simulink model "accTests"  (R2019a)
settings: Solver=VariableStepAuto  StartTime=0.0  StopTime=20  RelTol=1e-3
values from neighbouring files (symbols this model uses):
  ehMax = 3    [sim_parameters.m]
  ehMin = -100    [sim_parameters.m]
  g0 = 1/2*maxAccel*T^2 + maxAccel*T*t1 + + 1/2*maxAccel*t1^2 + 1/6*minJerk*t1^3 -      1/(2*minAccel)*(maxAccel*T + maxAccel*t1+ 1/2*minJerk*t1^2)^2    [safeHeadway.m]    (also in sim_parameters.m = ceil(g0*10)*1.1/10)
  h = figure()    [plotKinematicsFromSimulink.m]    (also in safeHeadway.m = T + t1 -      1/minAccel*(maxAccel*T + maxAccel*t1+1/2*minJe; sim_parameters.m = ceil(h*10)*1.1/10)
  Kd = K(1)    [SimulinkScenario.m]
  Ki = K(3)    [SimulinkScenario.m]
  Kp = K(2)    [SimulinkScenario.m]
  maxAcc = 4    [sim_parameters.m]
  maxJerk = 40    [sim_parameters.m]
  minAcc = -8    [sim_parameters.m]
  minJerk = -75    [sim_parameters.m]
  p = 10    [sim_parameters.m]
  vehMass = 2000    [sim_parameters.m]
  vLen = lf+lr    (= 3)    [sim_parameters.m]
libraries: autolibshared x5
settings Model: Creator=Fernando VM  LastModifiedBy=fvall
settings DataIOCC: ReturnWorkspaceOutputs=off
settings DebuggingCC: ArithmeticOperatorsInVariantConditions=warning

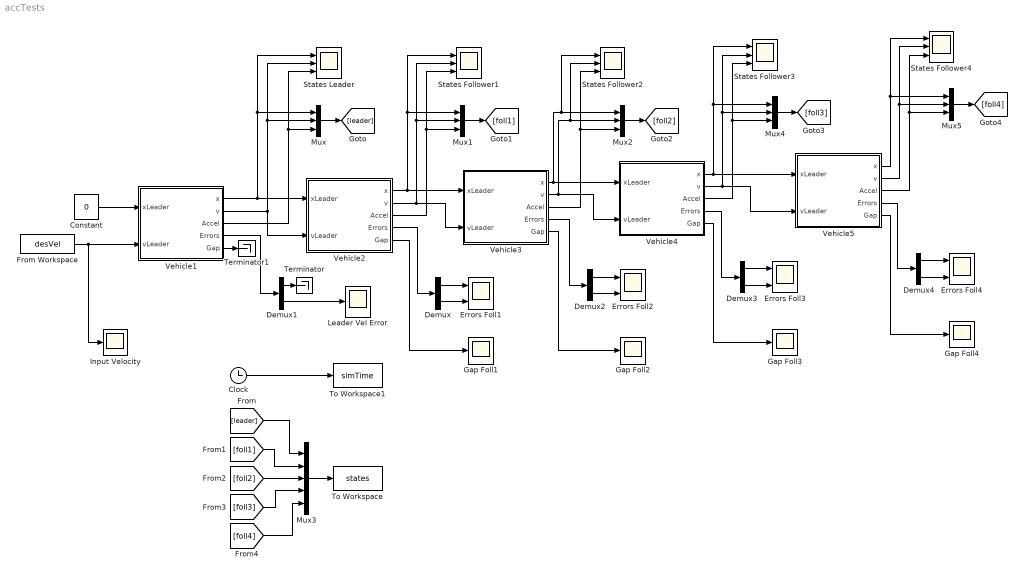
== system accTests ==
  Clock : Clock
  Constant : Constant  Value=0
  Demux{,1..4} (5 alike) : Demux  Outputs=2
  Errors Foll{1..4} (4 alike) : Scope  NumInputPorts=2
  From Workspace : FromWorkspace  VariableName=desVel  SampleTime=0
  Gap Foll{1..4} (4 alike) : Scope
  Input Velocity : Scope
  Leader Vel Error : Scope
  Mux{,1..2,4..5} (5 alike) : Mux  Inputs=3
  Mux3 : Mux  Inputs=5
  States Follower{1..4} (4 alike) : Scope  NumInputPorts=3
  States Leader : Scope  NumInputPorts=3
  Terminator : Terminator
  Terminator1 : Terminator
  To Workspace : ToWorkspace  VariableName=states  SampleTime=-1
  To Workspace1 : ToWorkspace  VariableName=simTime  SampleTime=-1
  Vehicle1 : Subsystem  mask{vehMass=vehMass, vLen=vLen, maxAcceleration=maxAcc, minAcceleration=minAcc, maxJerk=maxJerk, minJerk=minJerk, X_o=12.44, initVel=0, Kp=Kp, Kd=Kd, Ki=Ki, h=h, g0=g0, minHeadwayError=ehMin, maxHeadwayError=ehMax, velFilterGain=p}
      mask prompts: vehMass "Vehicle Mass"; vLen "Vehicle Length"; maxAcceleration "Max Acceleration"; minAcceleration "Min Acceleration"; maxJerk "Max Jerk"; minJerk "Min Jerk"; X_o "Initial Longitudinal Position"; initVel "Initial Longitudinal Velocity"; h "Time Headway"; g0 "Standstill Gap"; minHeadwayError "Min Headway Error"; maxHeadwayError "Max Headway Error"; velFilterGain "Velocity Filter Gain"
      mask DialogControl DescGroupVar Prompt: 3DOF Vehicle with ACC
      mask DialogControl DescTextVar Prompt: Vehicle with ACC. The vehicle model is Simulink's 3DOF single track vehicle body. The controller is a PID with constant headway including headway error saturation and filtered leader velocity.
      mask DialogControl ParameterGroupVar Prompt: Vehicle Parameters
      mask DialogControl Container3 Prompt: Controller Parameters
  Vehicle2 : Subsystem  mask{vehMass=vehMass, vLen=vLen, maxAcceleration=maxAcc, minAcceleration=minAcc, maxJerk=maxJerk, minJerk=minJerk, X_o=9.33, initVel=0, Kp=Kp, Kd=Kd, Ki=Ki, h=h, g0=g0, minHeadwayError=ehMin, maxHeadwayError=ehMax, velFilterGain=p}
      mask prompts: vehMass "Vehicle Mass"; vLen "Vehicle Length"; maxAcceleration "Max Acceleration"; minAcceleration "Min Acceleration"; maxJerk "Max Jerk"; minJerk "Min Jerk"; X_o "Initial Longitudinal Position"; initVel "Initial Longitudinal Velocity"; h "Time Headway"; g0 "Standstill Gap"; minHeadwayError "Min Headway Error"; maxHeadwayError "Max Headway Error"; velFilterGain "Velocity Filter Gain"
      mask DialogControl DescGroupVar Prompt: 3DOF Vehicle with ACC
      mask DialogControl DescTextVar Prompt: Vehicle with ACC. The vehicle model is Simulink's 3DOF single track vehicle body. The controller is a PID with constant headway including headway error saturation and filtered leader velocity.
      mask DialogControl ParameterGroupVar Prompt: Vehicle Parameters
      mask DialogControl Container3 Prompt: Controller Parameters
  Vehicle3 : Subsystem  mask{vehMass=vehMass, vLen=vLen, maxAcceleration=maxAcc, minAcceleration=minAcc, maxJerk=maxJerk, minJerk=minJerk, X_o=6.22, initVel=0, Kp=Kp, Kd=Kd, Ki=Ki, h=h, g0=g0, minHeadwayError=ehMin, maxHeadwayError=ehMax, velFilterGain=p}
      mask prompts: vehMass "Vehicle Mass"; vLen "Vehicle Length"; maxAcceleration "Max Acceleration"; minAcceleration "Min Acceleration"; maxJerk "Max Jerk"; minJerk "Min Jerk"; X_o "Initial Longitudinal Position"; initVel "Initial Longitudinal Velocity"; h "Time Headway"; g0 "Standstill Gap"; minHeadwayError "Min Headway Error"; maxHeadwayError "Max Headway Error"; velFilterGain "Velocity Filter Gain"
      mask DialogControl DescGroupVar Prompt: 3DOF Vehicle with ACC
      mask DialogControl DescTextVar Prompt: Vehicle with ACC. The vehicle model is Simulink's 3DOF single track vehicle body. The controller is a PID with constant headway including headway error saturation and filtered leader velocity.
      mask DialogControl ParameterGroupVar Prompt: Vehicle Parameters
      mask DialogControl Container3 Prompt: Controller Parameters
  Vehicle4 : Subsystem  mask{vehMass=vehMass, vLen=vLen, maxAcceleration=maxAcc, minAcceleration=minAcc, maxJerk=maxJerk, minJerk=minJerk, X_o=3.11, initVel=0, Kp=Kp, Kd=Kd, Ki=Ki, h=h, g0=g0, minHeadwayError=ehMin, maxHeadwayError=ehMax, velFilterGain=p}
      mask prompts: vehMass "Vehicle Mass"; vLen "Vehicle Length"; maxAcceleration "Max Acceleration"; minAcceleration "Min Acceleration"; maxJerk "Max Jerk"; minJerk "Min Jerk"; X_o "Initial Longitudinal Position"; initVel "Initial Longitudinal Velocity"; h "Time Headway"; g0 "Standstill Gap"; minHeadwayError "Min Headway Error"; maxHeadwayError "Max Headway Error"; velFilterGain "Velocity Filter Gain"
      mask DialogControl DescGroupVar Prompt: 3DOF Vehicle with ACC
      mask DialogControl DescTextVar Prompt: Vehicle with ACC. The vehicle model is Simulink's 3DOF single track vehicle body. The controller is a PID with constant headway including headway error saturation and filtered leader velocity.
      mask DialogControl ParameterGroupVar Prompt: Vehicle Parameters
      mask DialogControl Container3 Prompt: Controller Parameters
  Vehicle5 : Subsystem  mask{vehMass=vehMass, vLen=vLen, maxAcceleration=maxAcc, minAcceleration=minAcc, maxJerk=maxJerk, minJerk=minJerk, X_o=0, initVel=0, Kp=Kp, Kd=Kd, Ki=Ki, h=h, g0=g0, minHeadwayError=ehMin, maxHeadwayError=ehMax, velFilterGain=p}
      mask prompts: vehMass "Vehicle Mass"; vLen "Vehicle Length"; maxAcceleration "Max Acceleration"; minAcceleration "Min Acceleration"; maxJerk "Max Jerk"; minJerk "Min Jerk"; X_o "Initial Longitudinal Position"; initVel "Initial Longitudinal Velocity"; h "Time Headway"; g0 "Standstill Gap"; minHeadwayError "Min Headway Error"; maxHeadwayError "Max Headway Error"; velFilterGain "Velocity Filter Gain"
      mask DialogControl DescGroupVar Prompt: 3DOF Vehicle with ACC
      mask DialogControl DescTextVar Prompt: Vehicle with ACC. The vehicle model is Simulink's 3DOF single track vehicle body. The controller is a PID with constant headway including headway error saturation and filtered leader velocity.
      mask DialogControl ParameterGroupVar Prompt: Vehicle Parameters
      mask DialogControl Container3 Prompt: Controller Parameters
  wires:
  Vehicle2/5(Gap) -> Gap Foll1/1
  Vehicle5/3(Accel) -> Mux5/3, States Follower4/3
  Vehicle3/4(Errors) -> Demux2/1
  Vehicle3/1(x) -> Vehicle4/1(xLeader), Mux2/1, States Follower2/1
  Demux2/1 -> Errors Foll2/1
  Demux4/1 -> Errors Foll4/1
  Clock/1 -> To Workspace1/1
  Vehicle5/5(Gap) -> Gap Foll4/1
  Vehicle4/1(x) -> Vehicle5/1(xLeader), Mux4/1, States Follower3/1
  Vehicle4/3(Accel) -> Mux4/3, States Follower3/3
  Vehicle1/4(Errors) -> Demux1/1
  Demux/1 -> Errors Foll1/1
  Constant/1 -> Vehicle1/1(xLeader)
  Vehicle4/5(Gap) -> Gap Foll3/1
  Vehicle4/2(v) -> Vehicle5/2(vLeader), Mux4/2, States Follower3/2
  Mux4/1 -> [foll3]
  Vehicle2/1(x) -> Vehicle3/1(xLeader), Mux1/1, States Follower1/1
  Vehicle2/4(Errors) -> Demux/1
  Vehicle5/4(Errors) -> Demux4/1
  Vehicle3/2(v) -> Vehicle4/2(vLeader), Mux2/2, States Follower2/2
  Mux5/1 -> [foll4]
  Vehicle4/4(Errors) -> Demux3/1
  [foll1] -> Mux3/2
  Vehicle5/2(v) -> Mux5/2, States Follower4/2
  Demux4/2 -> Errors Foll4/2
  Vehicle1/1(x) -> Vehicle2/1(xLeader), States Leader/1, Mux/1
  Demux/2 -> Errors Foll1/2
  [foll3] -> Mux3/4
  [foll4] -> Mux3/5
  Mux3/1 -> To Workspace/1
  Mux2/1 -> [foll2]
  [leader] -> Mux3/1
  Mux1/1 -> [foll1]
  Mux/1 -> [leader]
  Demux2/2 -> Errors Foll2/2
  Vehicle2/2(v) -> Vehicle3/2(vLeader), Mux1/2, States Follower1/2
  [foll2] -> Mux3/3
  Vehicle2/3(Accel) -> Mux1/3, States Follower1/3
  Vehicle3/5(Gap) -> Gap Foll2/1
  Demux3/2 -> Errors Foll3/2
  Vehicle1/5(Gap) -> Terminator1/1
  Vehicle1/3(Accel) -> States Leader/3, Mux/3
  Demux1/2 -> Leader Vel Error/1
  Demux3/1 -> Errors Foll3/1
  Vehicle3/3(Accel) -> Mux2/3, States Follower2/3
  From Workspace/1 -> Input Velocity/1, Vehicle1/2(vLeader)
  Demux1/1 -> Terminator/1
  Vehicle1/2(v) -> Vehicle2/2(vLeader), Mux/2, States Leader/2
  Vehicle5/1(x) -> Mux5/1, States Follower4/1

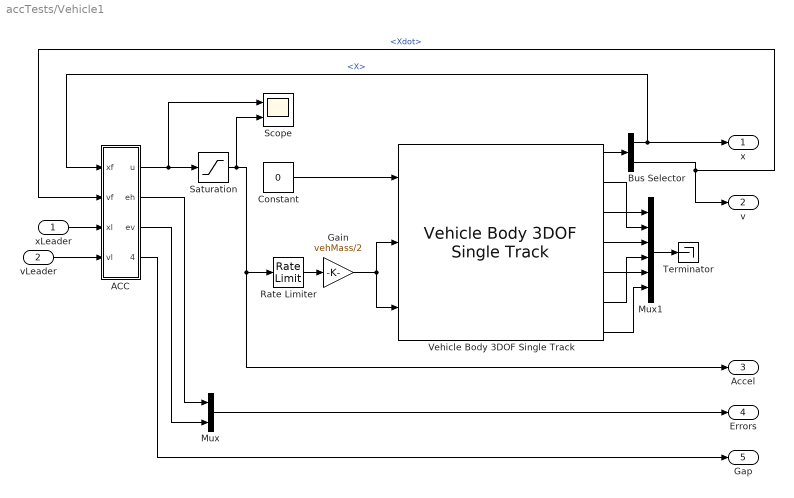
== system accTests/Vehicle1 ==
  xLeader : Inport
  vLeader : Inport  Port=2
  ACC : Subsystem
  Bus Selector : BusSelector  OutputSignals=InertFrm.RearAxl.Disp.X,InertFrm.RearAxl.Vel.Xdot
  Constant : Constant  Value=0
  Gain : Gain  Gain=vehMass/2
  Mux : Mux  Inputs=2
  Mux1 : Mux  Inputs=6
  Rate Limiter : RateLimiter  RisingSlewLimit=maxJerk  FallingSlewLimit=minJerk  SampleTimeMode=inherited
  Saturation : Saturate  UpperLimit=maxAcc  LowerLimit=minAcc
  Scope : Scope  NumInputPorts=2
  Terminator : Terminator
  Vehicle Body 3DOF Single Track : autolibshared/Vehicle Body 3DOF Single Track  trackMode=Single (bicycle)  inputMode=External longitudinal forces  frontSteerMode=on  rearSteerMode=off  windMode=off  muMode=off  extFMode=off  extMMode=off  extXo=off  extpsio=off  extxdoto=off  extro=off  extYo=off  extTamb=off  extydoto=off  aMode=2  NF=2  NR=2  m=vehMass  a=vLen/2  b=vLen/2  h=0.35  X_o=X_o  xdot_o=initVel  CalphaMode=off  sigmaMode=on  d=0  w=[1.4,1.4]  Cy_f=12e3  Cy_r=11e3  sigma_f=.1  sigma_r=.1  alpha_f_brk=[-.1 .1]  Cy_f_data=[-9e3 9e3]  alpha_r_brk=[-.1 .1]  Cy_r_data=[-9e3 9e3]  Y_o=0  ydot_o=0  Izz=4000  psi_o=0  r_o=0  Af=2  Cd=.3  Cl=.1  Cpm=.1  beta_w=[0:0.01:0.3]  Cs=[0:0.03:0.9]  Cym=[0:0.01:0.3]  Pabs=101325  Tair=273  g=9.81  mu=1  xdot_tol=.01  Fznom=5000  Fxtire_sat=7e4  Fytire_sat=7e4  longOff=0  latOff=0  vertOff=0  wrapAng=off
      settings: SourceProductName=Powertrain Blockset  SourceProductBaseCode=PW
  x : Outport
  v : Outport  Port=2
  Accel : Outport  Port=3
  Errors : Outport  Port=4
  Gap : Outport  Port=5
  wires:
  Bus Selector/2 -> ACC/2(vf), v/1  "<Xdot>"
  Bus Selector/1 -> x/1, ACC/1(xf)  "<X>"
  Saturation/1 -> Scope/2, Rate Limiter/1, Accel/1
  vLeader/1 -> ACC/4(vl)
  ACC/1(u) -> Scope/1, Saturation/1
  xLeader/1 -> ACC/3(xl)
  ACC/2(eh) -> Mux/1
  ACC/3(ev) -> Mux/2
  Mux/1 -> Errors/1
  Gain/1 -> Vehicle Body 3DOF Single Track/2, Vehicle Body 3DOF Single Track/3
  Constant/1 -> Vehicle Body 3DOF Single Track/1
  Vehicle Body 3DOF Single Track/1 -> Bus Selector/1
  Vehicle Body 3DOF Single Track/4 -> Mux1/3
  Vehicle Body 3DOF Single Track/3 -> Mux1/2
  Vehicle Body 3DOF Single Track/2 -> Mux1/1
  Vehicle Body 3DOF Single Track/5 -> Mux1/4
  Vehicle Body 3DOF Single Track/6 -> Mux1/5
  Vehicle Body 3DOF Single Track/7 -> Mux1/6
  Mux1/1 -> Terminator/1
  ACC/4(gap) -> Gap/1
  Rate Limiter/1 -> Gain/1

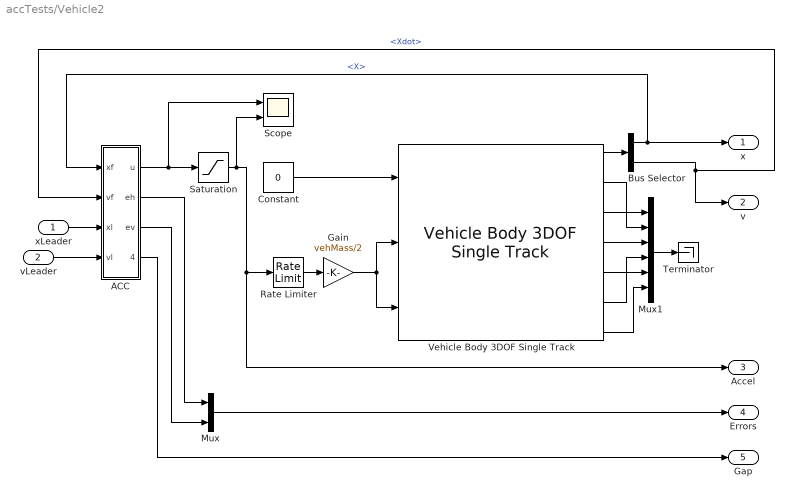
== system accTests/Vehicle2 ==
  xLeader : Inport
  vLeader : Inport  Port=2
  ACC : Subsystem
  Bus Selector : BusSelector  OutputSignals=InertFrm.RearAxl.Disp.X,InertFrm.RearAxl.Vel.Xdot
  Constant : Constant  Value=0
  Gain : Gain  Gain=vehMass/2
  Mux : Mux  Inputs=2
  Mux1 : Mux  Inputs=6
  Rate Limiter : RateLimiter  RisingSlewLimit=maxJerk  FallingSlewLimit=minJerk  SampleTimeMode=inherited
  Saturation : Saturate  UpperLimit=maxAcc  LowerLimit=minAcc
  Scope : Scope  NumInputPorts=2
  Terminator : Terminator
  Vehicle Body 3DOF Single Track : autolibshared/Vehicle Body 3DOF Single Track  trackMode=Single (bicycle)  inputMode=External longitudinal forces  frontSteerMode=on  rearSteerMode=off  windMode=off  muMode=off  extFMode=off  extMMode=off  extXo=off  extpsio=off  extxdoto=off  extro=off  extYo=off  extTamb=off  extydoto=off  aMode=2  NF=2  NR=2  m=vehMass  a=vLen/2  b=vLen/2  h=0.35  X_o=X_o  xdot_o=initVel  CalphaMode=off  sigmaMode=on  d=0  w=[1.4,1.4]  Cy_f=12e3  Cy_r=11e3  sigma_f=.1  sigma_r=.1  alpha_f_brk=[-.1 .1]  Cy_f_data=[-9e3 9e3]  alpha_r_brk=[-.1 .1]  Cy_r_data=[-9e3 9e3]  Y_o=0  ydot_o=0  Izz=4000  psi_o=0  r_o=0  Af=2  Cd=.3  Cl=.1  Cpm=.1  beta_w=[0:0.01:0.3]  Cs=[0:0.03:0.9]  Cym=[0:0.01:0.3]  Pabs=101325  Tair=273  g=9.81  mu=1  xdot_tol=.01  Fznom=5000  Fxtire_sat=7e4  Fytire_sat=7e4  longOff=0  latOff=0  vertOff=0  wrapAng=off
      settings: SourceProductName=Powertrain Blockset  SourceProductBaseCode=PW
  x : Outport
  v : Outport  Port=2
  Accel : Outport  Port=3
  Errors : Outport  Port=4
  Gap : Outport  Port=5
  wires:
  Bus Selector/2 -> ACC/2(vf), v/1  "<Xdot>"
  Bus Selector/1 -> x/1, ACC/1(xf)  "<X>"
  Saturation/1 -> Scope/2, Rate Limiter/1, Accel/1
  vLeader/1 -> ACC/4(vl)
  ACC/1(u) -> Scope/1, Saturation/1
  xLeader/1 -> ACC/3(xl)
  ACC/2(eh) -> Mux/1
  ACC/3(ev) -> Mux/2
  Mux/1 -> Errors/1
  Gain/1 -> Vehicle Body 3DOF Single Track/2, Vehicle Body 3DOF Single Track/3
  Constant/1 -> Vehicle Body 3DOF Single Track/1
  Vehicle Body 3DOF Single Track/1 -> Bus Selector/1
  Vehicle Body 3DOF Single Track/4 -> Mux1/3
  Vehicle Body 3DOF Single Track/3 -> Mux1/2
  Vehicle Body 3DOF Single Track/2 -> Mux1/1
  Vehicle Body 3DOF Single Track/5 -> Mux1/4
  Vehicle Body 3DOF Single Track/6 -> Mux1/5
  Vehicle Body 3DOF Single Track/7 -> Mux1/6
  Mux1/1 -> Terminator/1
  ACC/4(gap) -> Gap/1
  Rate Limiter/1 -> Gain/1

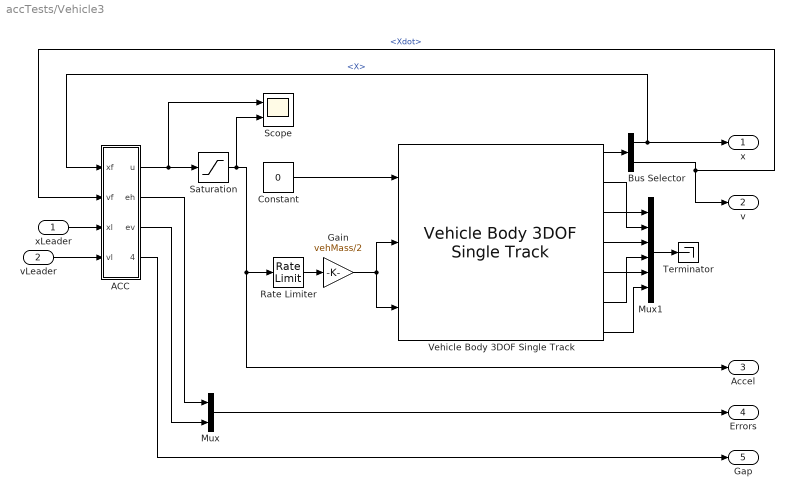
== system accTests/Vehicle3 ==
  xLeader : Inport
  vLeader : Inport  Port=2
  ACC : Subsystem
  Bus Selector : BusSelector  OutputSignals=InertFrm.RearAxl.Disp.X,InertFrm.RearAxl.Vel.Xdot
  Constant : Constant  Value=0
  Gain : Gain  Gain=vehMass/2
  Mux : Mux  Inputs=2
  Mux1 : Mux  Inputs=6
  Rate Limiter : RateLimiter  RisingSlewLimit=maxJerk  FallingSlewLimit=minJerk  SampleTimeMode=inherited
  Saturation : Saturate  UpperLimit=maxAcc  LowerLimit=minAcc
  Scope : Scope  NumInputPorts=2
  Terminator : Terminator
  Vehicle Body 3DOF Single Track : autolibshared/Vehicle Body 3DOF Single Track  trackMode=Single (bicycle)  inputMode=External longitudinal forces  frontSteerMode=on  rearSteerMode=off  windMode=off  muMode=off  extFMode=off  extMMode=off  extXo=off  extpsio=off  extxdoto=off  extro=off  extYo=off  extTamb=off  extydoto=off  aMode=2  NF=2  NR=2  m=vehMass  a=vLen/2  b=vLen/2  h=0.35  X_o=X_o  xdot_o=initVel  CalphaMode=off  sigmaMode=on  d=0  w=[1.4,1.4]  Cy_f=12e3  Cy_r=11e3  sigma_f=.1  sigma_r=.1  alpha_f_brk=[-.1 .1]  Cy_f_data=[-9e3 9e3]  alpha_r_brk=[-.1 .1]  Cy_r_data=[-9e3 9e3]  Y_o=0  ydot_o=0  Izz=4000  psi_o=0  r_o=0  Af=2  Cd=.3  Cl=.1  Cpm=.1  beta_w=[0:0.01:0.3]  Cs=[0:0.03:0.9]  Cym=[0:0.01:0.3]  Pabs=101325  Tair=273  g=9.81  mu=1  xdot_tol=.01  Fznom=5000  Fxtire_sat=7e4  Fytire_sat=7e4  longOff=0  latOff=0  vertOff=0  wrapAng=off
      settings: SourceProductName=Powertrain Blockset  SourceProductBaseCode=PW
  x : Outport
  v : Outport  Port=2
  Accel : Outport  Port=3
  Errors : Outport  Port=4
  Gap : Outport  Port=5
  wires:
  Bus Selector/2 -> ACC/2(vf), v/1  "<Xdot>"
  Bus Selector/1 -> x/1, ACC/1(xf)  "<X>"
  Saturation/1 -> Scope/2, Rate Limiter/1, Accel/1
  vLeader/1 -> ACC/4(vl)
  ACC/1(u) -> Scope/1, Saturation/1
  xLeader/1 -> ACC/3(xl)
  ACC/2(eh) -> Mux/1
  ACC/3(ev) -> Mux/2
  Mux/1 -> Errors/1
  Gain/1 -> Vehicle Body 3DOF Single Track/2, Vehicle Body 3DOF Single Track/3
  Constant/1 -> Vehicle Body 3DOF Single Track/1
  Vehicle Body 3DOF Single Track/1 -> Bus Selector/1
  Vehicle Body 3DOF Single Track/4 -> Mux1/3
  Vehicle Body 3DOF Single Track/3 -> Mux1/2
  Vehicle Body 3DOF Single Track/2 -> Mux1/1
  Vehicle Body 3DOF Single Track/5 -> Mux1/4
  Vehicle Body 3DOF Single Track/6 -> Mux1/5
  Vehicle Body 3DOF Single Track/7 -> Mux1/6
  Mux1/1 -> Terminator/1
  ACC/4(gap) -> Gap/1
  Rate Limiter/1 -> Gain/1

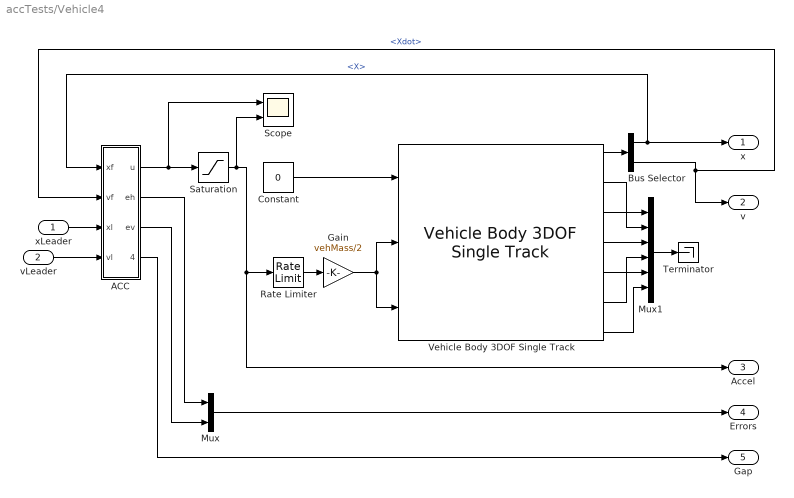
== system accTests/Vehicle4 ==
  xLeader : Inport
  vLeader : Inport  Port=2
  ACC : Subsystem
  Bus Selector : BusSelector  OutputSignals=InertFrm.RearAxl.Disp.X,InertFrm.RearAxl.Vel.Xdot
  Constant : Constant  Value=0
  Gain : Gain  Gain=vehMass/2
  Mux : Mux  Inputs=2
  Mux1 : Mux  Inputs=6
  Rate Limiter : RateLimiter  RisingSlewLimit=maxJerk  FallingSlewLimit=minJerk  SampleTimeMode=inherited
  Saturation : Saturate  UpperLimit=maxAcc  LowerLimit=minAcc
  Scope : Scope  NumInputPorts=2
  Terminator : Terminator
  Vehicle Body 3DOF Single Track : autolibshared/Vehicle Body 3DOF Single Track  trackMode=Single (bicycle)  inputMode=External longitudinal forces  frontSteerMode=on  rearSteerMode=off  windMode=off  muMode=off  extFMode=off  extMMode=off  extXo=off  extpsio=off  extxdoto=off  extro=off  extYo=off  extTamb=off  extydoto=off  aMode=2  NF=2  NR=2  m=vehMass  a=vLen/2  b=vLen/2  h=0.35  X_o=X_o  xdot_o=initVel  CalphaMode=off  sigmaMode=on  d=0  w=[1.4,1.4]  Cy_f=12e3  Cy_r=11e3  sigma_f=.1  sigma_r=.1  alpha_f_brk=[-.1 .1]  Cy_f_data=[-9e3 9e3]  alpha_r_brk=[-.1 .1]  Cy_r_data=[-9e3 9e3]  Y_o=0  ydot_o=0  Izz=4000  psi_o=0  r_o=0  Af=2  Cd=.3  Cl=.1  Cpm=.1  beta_w=[0:0.01:0.3]  Cs=[0:0.03:0.9]  Cym=[0:0.01:0.3]  Pabs=101325  Tair=273  g=9.81  mu=1  xdot_tol=.01  Fznom=5000  Fxtire_sat=7e4  Fytire_sat=7e4  longOff=0  latOff=0  vertOff=0  wrapAng=off
      settings: SourceProductName=Powertrain Blockset  SourceProductBaseCode=PW
  x : Outport
  v : Outport  Port=2
  Accel : Outport  Port=3
  Errors : Outport  Port=4
  Gap : Outport  Port=5
  wires:
  Bus Selector/2 -> ACC/2(vf), v/1  "<Xdot>"
  Bus Selector/1 -> x/1, ACC/1(xf)  "<X>"
  Saturation/1 -> Scope/2, Rate Limiter/1, Accel/1
  vLeader/1 -> ACC/4(vl)
  ACC/1(u) -> Scope/1, Saturation/1
  xLeader/1 -> ACC/3(xl)
  ACC/2(eh) -> Mux/1
  ACC/3(ev) -> Mux/2
  Mux/1 -> Errors/1
  Gain/1 -> Vehicle Body 3DOF Single Track/2, Vehicle Body 3DOF Single Track/3
  Constant/1 -> Vehicle Body 3DOF Single Track/1
  Vehicle Body 3DOF Single Track/1 -> Bus Selector/1
  Vehicle Body 3DOF Single Track/4 -> Mux1/3
  Vehicle Body 3DOF Single Track/3 -> Mux1/2
  Vehicle Body 3DOF Single Track/2 -> Mux1/1
  Vehicle Body 3DOF Single Track/5 -> Mux1/4
  Vehicle Body 3DOF Single Track/6 -> Mux1/5
  Vehicle Body 3DOF Single Track/7 -> Mux1/6
  Mux1/1 -> Terminator/1
  ACC/4(gap) -> Gap/1
  Rate Limiter/1 -> Gain/1

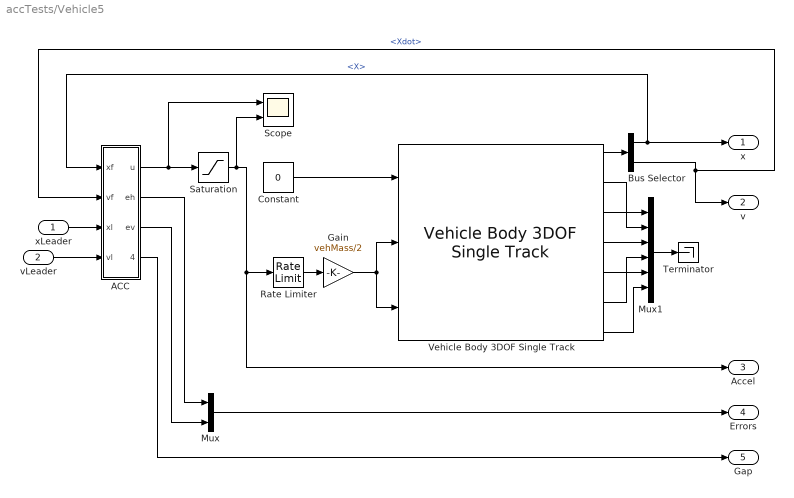
== system accTests/Vehicle5 ==
  xLeader : Inport
  vLeader : Inport  Port=2
  ACC : Subsystem
  Bus Selector : BusSelector  OutputSignals=InertFrm.RearAxl.Disp.X,InertFrm.RearAxl.Vel.Xdot
  Constant : Constant  Value=0
  Gain : Gain  Gain=vehMass/2
  Mux : Mux  Inputs=2
  Mux1 : Mux  Inputs=6
  Rate Limiter : RateLimiter  RisingSlewLimit=maxJerk  FallingSlewLimit=minJerk  SampleTimeMode=inherited
  Saturation : Saturate  UpperLimit=maxAcc  LowerLimit=minAcc
  Scope : Scope  NumInputPorts=2
  Terminator : Terminator
  Vehicle Body 3DOF Single Track : autolibshared/Vehicle Body 3DOF Single Track  trackMode=Single (bicycle)  inputMode=External longitudinal forces  frontSteerMode=on  rearSteerMode=off  windMode=off  muMode=off  extFMode=off  extMMode=off  extXo=off  extpsio=off  extxdoto=off  extro=off  extYo=off  extTamb=off  extydoto=off  aMode=2  NF=2  NR=2  m=vehMass  a=vLen/2  b=vLen/2  h=0.35  X_o=X_o  xdot_o=initVel  CalphaMode=off  sigmaMode=on  d=0  w=[1.4,1.4]  Cy_f=12e3  Cy_r=11e3  sigma_f=.1  sigma_r=.1  alpha_f_brk=[-.1 .1]  Cy_f_data=[-9e3 9e3]  alpha_r_brk=[-.1 .1]  Cy_r_data=[-9e3 9e3]  Y_o=0  ydot_o=0  Izz=4000  psi_o=0  r_o=0  Af=2  Cd=.3  Cl=.1  Cpm=.1  beta_w=[0:0.01:0.3]  Cs=[0:0.03:0.9]  Cym=[0:0.01:0.3]  Pabs=101325  Tair=273  g=9.81  mu=1  xdot_tol=.01  Fznom=5000  Fxtire_sat=7e4  Fytire_sat=7e4  longOff=0  latOff=0  vertOff=0  wrapAng=off
      settings: SourceProductName=Powertrain Blockset  SourceProductBaseCode=PW
  x : Outport
  v : Outport  Port=2
  Accel : Outport  Port=3
  Errors : Outport  Port=4
  Gap : Outport  Port=5
  wires:
  Bus Selector/2 -> ACC/2(vf), v/1  "<Xdot>"
  Bus Selector/1 -> x/1, ACC/1(xf)  "<X>"
  Saturation/1 -> Scope/2, Rate Limiter/1, Accel/1
  vLeader/1 -> ACC/4(vl)
  ACC/1(u) -> Scope/1, Saturation/1
  xLeader/1 -> ACC/3(xl)
  ACC/2(eh) -> Mux/1
  ACC/3(ev) -> Mux/2
  Mux/1 -> Errors/1
  Gain/1 -> Vehicle Body 3DOF Single Track/2, Vehicle Body 3DOF Single Track/3
  Constant/1 -> Vehicle Body 3DOF Single Track/1
  Vehicle Body 3DOF Single Track/1 -> Bus Selector/1
  Vehicle Body 3DOF Single Track/4 -> Mux1/3
  Vehicle Body 3DOF Single Track/3 -> Mux1/2
  Vehicle Body 3DOF Single Track/2 -> Mux1/1
  Vehicle Body 3DOF Single Track/5 -> Mux1/4
  Vehicle Body 3DOF Single Track/6 -> Mux1/5
  Vehicle Body 3DOF Single Track/7 -> Mux1/6
  Mux1/1 -> Terminator/1
  ACC/4(gap) -> Gap/1
  Rate Limiter/1 -> Gain/1

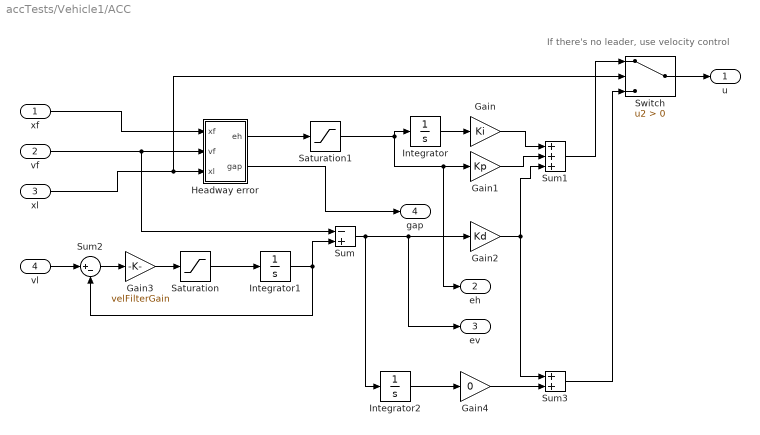
== system accTests/Vehicle1/ACC ==
  note: If there's no leader, use velocity control
  xf : Inport
  vf : Inport  Port=2
  xl : Inport  Port=3
  vl : Inport  Port=4
  Gain : Gain  Gain=Ki
  Gain1 : Gain  Gain=Kp
  Gain2 : Gain  Gain=Kd
  Gain3 : Gain  Gain=velFilterGain
  Gain4 : Gain  Gain=0
  Headway error : Subsystem  mask{vLen=vLen, g0=g0, h=h}
      mask prompts: vLen "Vehicle Length"; g0 "Standstill Gap"; h "Time Headway"
      mask init:
      | vLen >= 0;
      | g0 >= 0;
      | h >= 0;
  Integrator : Integrator
  Integrator1 : Integrator  InitialCondition=initVel
  Integrator2 : Integrator
  Saturation : Saturate  UpperLimit=maxAcceleration  LowerLimit=minAcceleration
  Saturation1 : Saturate  UpperLimit=maxHeadwayError  LowerLimit=minHeadwayError
  Sum : Sum  Inputs=-+
  Sum1 : Sum  Inputs=+++
  Sum2 : Sum  Inputs=|+-
  Sum3 : Sum
  Switch : Switch  Criteria=u2 > Threshold
  u : Outport
  eh : Outport  Port=2
  ev : Outport  Port=3
  gap : Outport  Port=4
  wires:
  Headway error/1(eh) -> Saturation1/1
  vf/1 -> Sum/1, Headway error/2(vf)
  Gain2/1 -> Sum3/1, Sum1/3
  Gain1/1 -> Sum1/2
  Gain/1 -> Sum1/1
  Integrator/1 -> Gain/1
  xl/1 -> Switch/2, Headway error/3(xl)
  xf/1 -> Headway error/1(xf)
  Gain3/1 -> Saturation/1
  Saturation/1 -> Integrator1/1
  Integrator1/1 -> Sum2/2, Sum/2
  vl/1 -> Sum2/1
  Sum2/1 -> Gain3/1
  Saturation1/1 -> eh/1, Gain1/1, Integrator/1
  Headway error/2("gap ") -> gap/1
  Integrator2/1 -> Gain4/1
  Gain4/1 -> Sum3/2
  Switch/1 -> u/1
  Sum1/1 -> Switch/1
  Sum3/1 -> Switch/3
  Sum/1 -> Integrator2/1, ev/1, Gain2/1

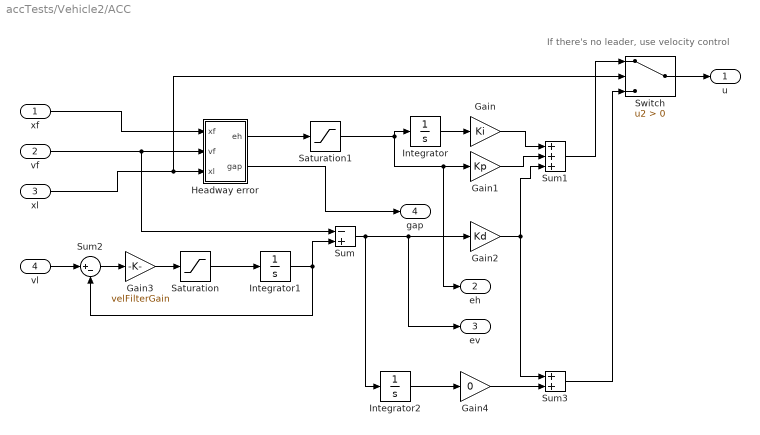
== system accTests/Vehicle2/ACC ==
  note: If there's no leader, use velocity control
  xf : Inport
  vf : Inport  Port=2
  xl : Inport  Port=3
  vl : Inport  Port=4
  Gain : Gain  Gain=Ki
  Gain1 : Gain  Gain=Kp
  Gain2 : Gain  Gain=Kd
  Gain3 : Gain  Gain=velFilterGain
  Gain4 : Gain  Gain=0
  Headway error : Subsystem  mask{vLen=vLen, g0=g0, h=h}
      mask prompts: vLen "Vehicle Length"; g0 "Standstill Gap"; h "Time Headway"
      mask init:
      | vLen >= 0;
      | g0 >= 0;
      | h >= 0;
  Integrator : Integrator
  Integrator1 : Integrator  InitialCondition=initVel
  Integrator2 : Integrator
  Saturation : Saturate  UpperLimit=maxAcceleration  LowerLimit=minAcceleration
  Saturation1 : Saturate  UpperLimit=maxHeadwayError  LowerLimit=minHeadwayError
  Sum : Sum  Inputs=-+
  Sum1 : Sum  Inputs=+++
  Sum2 : Sum  Inputs=|+-
  Sum3 : Sum
  Switch : Switch  Criteria=u2 > Threshold
  u : Outport
  eh : Outport  Port=2
  ev : Outport  Port=3
  gap : Outport  Port=4
  wires:
  Headway error/1(eh) -> Saturation1/1
  vf/1 -> Sum/1, Headway error/2(vf)
  Gain2/1 -> Sum3/1, Sum1/3
  Gain1/1 -> Sum1/2
  Gain/1 -> Sum1/1
  Integrator/1 -> Gain/1
  xl/1 -> Switch/2, Headway error/3(xl)
  xf/1 -> Headway error/1(xf)
  Gain3/1 -> Saturation/1
  Saturation/1 -> Integrator1/1
  Integrator1/1 -> Sum2/2, Sum/2
  vl/1 -> Sum2/1
  Sum2/1 -> Gain3/1
  Saturation1/1 -> eh/1, Gain1/1, Integrator/1
  Headway error/2("gap ") -> gap/1
  Integrator2/1 -> Gain4/1
  Gain4/1 -> Sum3/2
  Switch/1 -> u/1
  Sum1/1 -> Switch/1
  Sum3/1 -> Switch/3
  Sum/1 -> Integrator2/1, ev/1, Gain2/1

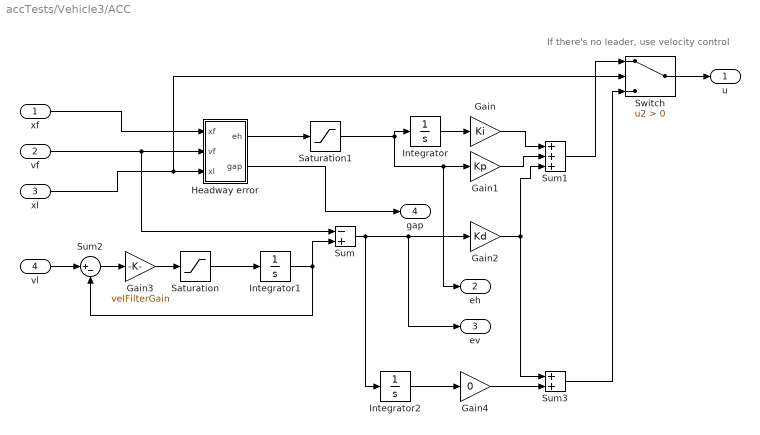
== system accTests/Vehicle3/ACC ==
  note: If there's no leader, use velocity control
  xf : Inport
  vf : Inport  Port=2
  xl : Inport  Port=3
  vl : Inport  Port=4
  Gain : Gain  Gain=Ki
  Gain1 : Gain  Gain=Kp
  Gain2 : Gain  Gain=Kd
  Gain3 : Gain  Gain=velFilterGain
  Gain4 : Gain  Gain=0
  Headway error : Subsystem  mask{vLen=vLen, g0=g0, h=h}
      mask prompts: vLen "Vehicle Length"; g0 "Standstill Gap"; h "Time Headway"
      mask init:
      | vLen >= 0;
      | g0 >= 0;
      | h >= 0;
  Integrator : Integrator
  Integrator1 : Integrator  InitialCondition=initVel
  Integrator2 : Integrator
  Saturation : Saturate  UpperLimit=maxAcceleration  LowerLimit=minAcceleration
  Saturation1 : Saturate  UpperLimit=maxHeadwayError  LowerLimit=minHeadwayError
  Sum : Sum  Inputs=-+
  Sum1 : Sum  Inputs=+++
  Sum2 : Sum  Inputs=|+-
  Sum3 : Sum
  Switch : Switch  Criteria=u2 > Threshold
  u : Outport
  eh : Outport  Port=2
  ev : Outport  Port=3
  gap : Outport  Port=4
  wires:
  Headway error/1(eh) -> Saturation1/1
  vf/1 -> Sum/1, Headway error/2(vf)
  Gain2/1 -> Sum3/1, Sum1/3
  Gain1/1 -> Sum1/2
  Gain/1 -> Sum1/1
  Integrator/1 -> Gain/1
  xl/1 -> Switch/2, Headway error/3(xl)
  xf/1 -> Headway error/1(xf)
  Gain3/1 -> Saturation/1
  Saturation/1 -> Integrator1/1
  Integrator1/1 -> Sum2/2, Sum/2
  vl/1 -> Sum2/1
  Sum2/1 -> Gain3/1
  Saturation1/1 -> eh/1, Gain1/1, Integrator/1
  Headway error/2("gap ") -> gap/1
  Integrator2/1 -> Gain4/1
  Gain4/1 -> Sum3/2
  Switch/1 -> u/1
  Sum1/1 -> Switch/1
  Sum3/1 -> Switch/3
  Sum/1 -> Integrator2/1, ev/1, Gain2/1

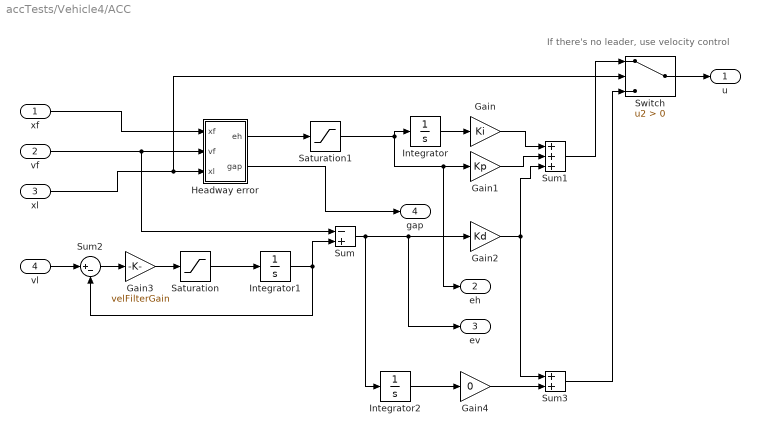
== system accTests/Vehicle4/ACC ==
  note: If there's no leader, use velocity control
  xf : Inport
  vf : Inport  Port=2
  xl : Inport  Port=3
  vl : Inport  Port=4
  Gain : Gain  Gain=Ki
  Gain1 : Gain  Gain=Kp
  Gain2 : Gain  Gain=Kd
  Gain3 : Gain  Gain=velFilterGain
  Gain4 : Gain  Gain=0
  Headway error : Subsystem  mask{vLen=vLen, g0=g0, h=h}
      mask prompts: vLen "Vehicle Length"; g0 "Standstill Gap"; h "Time Headway"
      mask init:
      | vLen >= 0;
      | g0 >= 0;
      | h >= 0;
  Integrator : Integrator
  Integrator1 : Integrator  InitialCondition=initVel
  Integrator2 : Integrator
  Saturation : Saturate  UpperLimit=maxAcceleration  LowerLimit=minAcceleration
  Saturation1 : Saturate  UpperLimit=maxHeadwayError  LowerLimit=minHeadwayError
  Sum : Sum  Inputs=-+
  Sum1 : Sum  Inputs=+++
  Sum2 : Sum  Inputs=|+-
  Sum3 : Sum
  Switch : Switch  Criteria=u2 > Threshold
  u : Outport
  eh : Outport  Port=2
  ev : Outport  Port=3
  gap : Outport  Port=4
  wires:
  Headway error/1(eh) -> Saturation1/1
  vf/1 -> Sum/1, Headway error/2(vf)
  Gain2/1 -> Sum3/1, Sum1/3
  Gain1/1 -> Sum1/2
  Gain/1 -> Sum1/1
  Integrator/1 -> Gain/1
  xl/1 -> Switch/2, Headway error/3(xl)
  xf/1 -> Headway error/1(xf)
  Gain3/1 -> Saturation/1
  Saturation/1 -> Integrator1/1
  Integrator1/1 -> Sum2/2, Sum/2
  vl/1 -> Sum2/1
  Sum2/1 -> Gain3/1
  Saturation1/1 -> eh/1, Gain1/1, Integrator/1
  Headway error/2("gap ") -> gap/1
  Integrator2/1 -> Gain4/1
  Gain4/1 -> Sum3/2
  Switch/1 -> u/1
  Sum1/1 -> Switch/1
  Sum3/1 -> Switch/3
  Sum/1 -> Integrator2/1, ev/1, Gain2/1

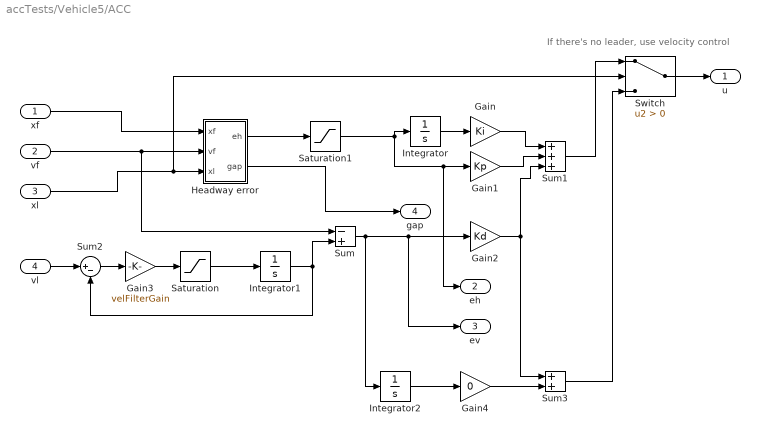
== system accTests/Vehicle5/ACC ==
  note: If there's no leader, use velocity control
  xf : Inport
  vf : Inport  Port=2
  xl : Inport  Port=3
  vl : Inport  Port=4
  Gain : Gain  Gain=Ki
  Gain1 : Gain  Gain=Kp
  Gain2 : Gain  Gain=Kd
  Gain3 : Gain  Gain=velFilterGain
  Gain4 : Gain  Gain=0
  Headway error : Subsystem  mask{vLen=vLen, g0=g0, h=h}
      mask prompts: vLen "Vehicle Length"; g0 "Standstill Gap"; h "Time Headway"
      mask init:
      | vLen >= 0;
      | g0 >= 0;
      | h >= 0;
  Integrator : Integrator
  Integrator1 : Integrator  InitialCondition=initVel
  Integrator2 : Integrator
  Saturation : Saturate  UpperLimit=maxAcceleration  LowerLimit=minAcceleration
  Saturation1 : Saturate  UpperLimit=maxHeadwayError  LowerLimit=minHeadwayError
  Sum : Sum  Inputs=-+
  Sum1 : Sum  Inputs=+++
  Sum2 : Sum  Inputs=|+-
  Sum3 : Sum
  Switch : Switch  Criteria=u2 > Threshold
  u : Outport
  eh : Outport  Port=2
  ev : Outport  Port=3
  gap : Outport  Port=4
  wires:
  Headway error/1(eh) -> Saturation1/1
  vf/1 -> Sum/1, Headway error/2(vf)
  Gain2/1 -> Sum3/1, Sum1/3
  Gain1/1 -> Sum1/2
  Gain/1 -> Sum1/1
  Integrator/1 -> Gain/1
  xl/1 -> Switch/2, Headway error/3(xl)
  xf/1 -> Headway error/1(xf)
  Gain3/1 -> Saturation/1
  Saturation/1 -> Integrator1/1
  Integrator1/1 -> Sum2/2, Sum/2
  vl/1 -> Sum2/1
  Sum2/1 -> Gain3/1
  Saturation1/1 -> eh/1, Gain1/1, Integrator/1
  Headway error/2("gap ") -> gap/1
  Integrator2/1 -> Gain4/1
  Gain4/1 -> Sum3/2
  Switch/1 -> u/1
  Sum1/1 -> Switch/1
  Sum3/1 -> Switch/3
  Sum/1 -> Integrator2/1, ev/1, Gain2/1

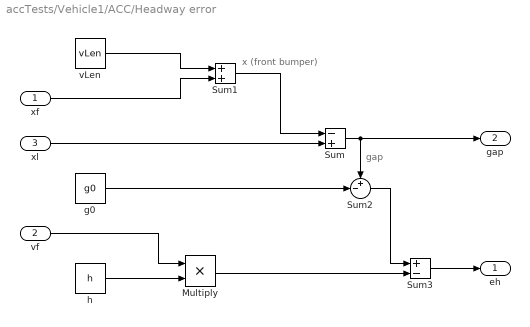
== system accTests/Vehicle1/ACC/Headway error ==
  note: gap
  note: x (front bumper)
  xf : Inport
  vf : Inport  Port=2
  xl : Inport  Port=3
  Multiply : Product
  Sum : Sum  Inputs=-+
  Sum1 : Sum
  Sum2 : Sum  Inputs=+-|
  Sum3 : Sum  Inputs=+-
  g0 : Constant  Value=g0
  h : Constant  Value=h
  vLen : Constant  Value=vLen
  eh : Outport
  "gap " : Outport  Port=2
  wires:
  vLen/1 -> Sum1/1
  Multiply/1 -> Sum3/2
  g0/1 -> Sum2/2
  Sum2/1 -> Sum3/1
  Sum/1 -> "gap "/1, Sum2/1
  xf/1 -> Sum1/2
  Sum3/1 -> eh/1
  vf/1 -> Multiply/1
  h/1 -> Multiply/2
  Sum1/1 -> Sum/1
  xl/1 -> Sum/2

== system accTests/Vehicle2/ACC/Headway error ==
  note: gap
  note: x (front bumper)
  xf : Inport
  vf : Inport  Port=2
  xl : Inport  Port=3
  Multiply : Product
  Sum : Sum  Inputs=-+
  Sum1 : Sum
  Sum2 : Sum  Inputs=+-|
  Sum3 : Sum  Inputs=+-
  g0 : Constant  Value=g0
  h : Constant  Value=h
  vLen : Constant  Value=vLen
  eh : Outport
  "gap " : Outport  Port=2
  wires:
  vLen/1 -> Sum1/1
  Multiply/1 -> Sum3/2
  g0/1 -> Sum2/2
  Sum2/1 -> Sum3/1
  Sum/1 -> "gap "/1, Sum2/1
  xf/1 -> Sum1/2
  Sum3/1 -> eh/1
  vf/1 -> Multiply/1
  h/1 -> Multiply/2
  Sum1/1 -> Sum/1
  xl/1 -> Sum/2

== system accTests/Vehicle3/ACC/Headway error ==
  note: gap
  note: x (front bumper)
  xf : Inport
  vf : Inport  Port=2
  xl : Inport  Port=3
  Multiply : Product
  Sum : Sum  Inputs=-+
  Sum1 : Sum
  Sum2 : Sum  Inputs=+-|
  Sum3 : Sum  Inputs=+-
  g0 : Constant  Value=g0
  h : Constant  Value=h
  vLen : Constant  Value=vLen
  eh : Outport
  "gap " : Outport  Port=2
  wires:
  vLen/1 -> Sum1/1
  Multiply/1 -> Sum3/2
  g0/1 -> Sum2/2
  Sum2/1 -> Sum3/1
  Sum/1 -> "gap "/1, Sum2/1
  xf/1 -> Sum1/2
  Sum3/1 -> eh/1
  vf/1 -> Multiply/1
  h/1 -> Multiply/2
  Sum1/1 -> Sum/1
  xl/1 -> Sum/2

== system accTests/Vehicle4/ACC/Headway error ==
  note: gap
  note: x (front bumper)
  xf : Inport
  vf : Inport  Port=2
  xl : Inport  Port=3
  Multiply : Product
  Sum : Sum  Inputs=-+
  Sum1 : Sum
  Sum2 : Sum  Inputs=+-|
  Sum3 : Sum  Inputs=+-
  g0 : Constant  Value=g0
  h : Constant  Value=h
  vLen : Constant  Value=vLen
  eh : Outport
  "gap " : Outport  Port=2
  wires:
  vLen/1 -> Sum1/1
  Multiply/1 -> Sum3/2
  g0/1 -> Sum2/2
  Sum2/1 -> Sum3/1
  Sum/1 -> "gap "/1, Sum2/1
  xf/1 -> Sum1/2
  Sum3/1 -> eh/1
  vf/1 -> Multiply/1
  h/1 -> Multiply/2
  Sum1/1 -> Sum/1
  xl/1 -> Sum/2

== system accTests/Vehicle5/ACC/Headway error ==
  note: gap
  note: x (front bumper)
  xf : Inport
  vf : Inport  Port=2
  xl : Inport  Port=3
  Multiply : Product
  Sum : Sum  Inputs=-+
  Sum1 : Sum
  Sum2 : Sum  Inputs=+-|
  Sum3 : Sum  Inputs=+-
  g0 : Constant  Value=g0
  h : Constant  Value=h
  vLen : Constant  Value=vLen
  eh : Outport
  "gap " : Outport  Port=2
  wires:
  vLen/1 -> Sum1/1
  Multiply/1 -> Sum3/2
  g0/1 -> Sum2/2
  Sum2/1 -> Sum3/1
  Sum/1 -> "gap "/1, Sum2/1
  xf/1 -> Sum1/2
  Sum3/1 -> eh/1
  vf/1 -> Multiply/1
  h/1 -> Multiply/2
  Sum1/1 -> Sum/1
  xl/1 -> Sum/2
